simulink model "SF034A_AssiPahFwl"  (R2013b)
settings: Solver=FixedStepDiscrete  SolverMode=SingleTasking  StartTime=0.0  StopTime=1  FixedStep=0.002  RelTol=1e-3
values from neighbouring files (symbols this model uses):
  ARCHGLBPRM_2MILLISEC_SEC_F32 = DataDict.Constant    [SF034A_AssiPahFwl_DataDict.m]
  AssiPahFwlDiRcvr = DataDict.Calibration    [SF034A_AssiPahFwl_DataDict.m]
  AssiPahFwlHysCmpLim = DataDict.Calibration    [SF034A_AssiPahFwl_DataDict.m]
  AssiPahFwlRestoreThd = DataDict.Calibration    [SF034A_AssiPahFwl_DataDict.m]
  BasAssiPahFwlOverLimDiagcFailStep = DataDict.Calibration    [SF034A_AssiPahFwl_DataDict.m]
  BasAssiPahFwlOverLimDiagcPassStep = DataDict.Calibration    [SF034A_AssiPahFwl_DataDict.m]
  BASASSIREACHED_CNT_U08 = DataDict.Constant    [SF034A_AssiPahFwl_DataDict.m]
  HiFrqAssiPahFwlOverLimDiagcFailStep = DataDict.Calibration    [SF034A_AssiPahFwl_DataDict.m]
  HiFrqAssiPahFwlOverLimDiagcPassStep = DataDict.Calibration    [SF034A_AssiPahFwl_DataDict.m]
  HIFRQASSIREACHED_CNT_U08 = DataDict.Constant    [SF034A_AssiPahFwl_DataDict.m]
undefined symbols (not defined in the file or in its folder): MfgEnaSt1, NtcNr1, NtcSts1, sigbuilder_block, SigQlfr1
libraries: simulink x23, Fil x8, NxtrLim x5, FixdToFloat x5, BilnrIntrpnMplX x4, FloatToFixd x4, NxtrAbslt x2, LnrIntrpn x1, NxtrSign x1
(part 2 of 3)

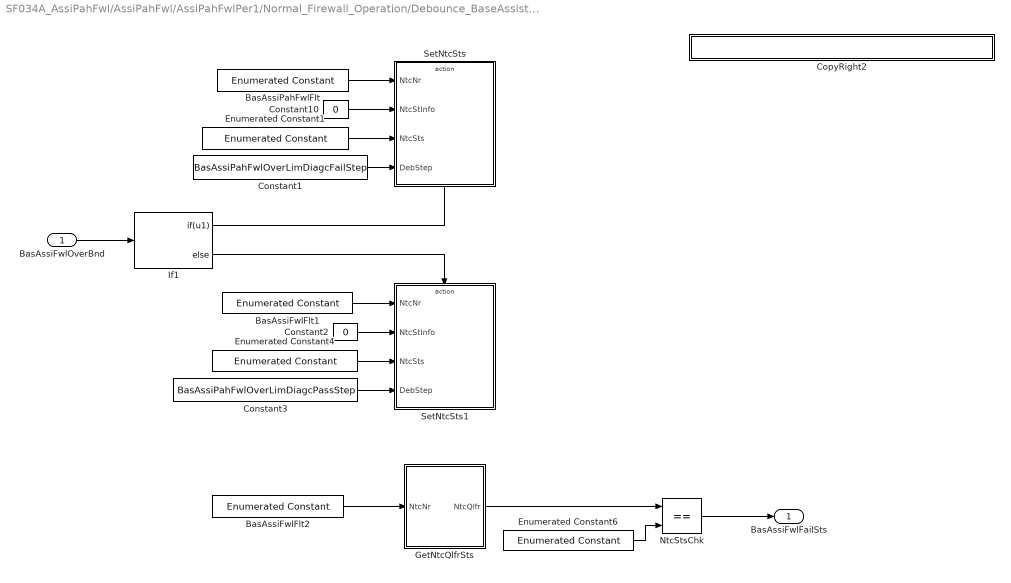
== system SF034A_AssiPahFwl/AssiPahFwl/AssiPahFwlPer1/Normal_Firewall_Operation/Debounce_BaseAssist_Overboundary ==
  BasAssiFwlOverBnd : Inport
  BasAssiFwlFlt1 : simulink/Sources/Enumerated Constant  RequirementInfo={} %GIDa_2f1a8232_f62b_44d9_9001_15c30141b4fe  OutDataTypeStr=Enum: NtcNr1  Value=NtcNr1.NTCNR_0X0D3  SampleTime=inf
  BasAssiFwlFlt2 : simulink/Sources/Enumerated Constant  RequirementInfo={} %GIDa_a465f244_f927_4bf7_a173_7ecad0b77852  OutDataTypeStr=Enum: NtcNr1  Value=NtcNr1.NTCNR_0X0D3  SampleTime=inf
  BasAssiPahFwlFlt : simulink/Sources/Enumerated Constant  RequirementInfo={} %GIDa_799d57aa_42cf_4c29_8873_5e7f7c5dd1ab  OutDataTypeStr=Enum: NtcNr1  Value=NtcNr1.NTCNR_0X0D3  SampleTime=inf
  Constant1 : Constant  Value=BasAssiPahFwlOverLimDiagcFailStep  OutDataTypeStr=uint16
  Constant10 : Constant  Value=0
  Constant2 : Constant  Value=0
  Constant3 : Constant  Value=BasAssiPahFwlOverLimDiagcPassStep  OutDataTypeStr=uint16
  CopyRight2 : Subsystem  Description=|  mask(Copyright Information){none=on}
      | Copyright info block.                                               
      |                                                                     
      | Place copyright information at the top of every subsystem in design.
      mask prompts: none "No parameters"
      mask help: Place copyright information at the top of every subsystem in design.
      mask Display:
      | NxtrConf = 'Nexteer Confidential';
      | 
      | sys = bdroot; %handle for the current model ("system")
      | first = get_param(sys,'Created');
      | first = first(end-3:end);  %year is last four digits
      | 
      | last = get_param(sys,'LastModifiedDate');
      | if isempty(last)
      |     last = datestr(now,'yyyy');
      | else
      |     last = last(end-3:end);
      | end
      | 
      | if strcmp(first,last)
      |     fprintf('%s -- Copyright %s Nexteer',NxtrConf,first)
      | else
      |     fprintf('%s -- %s%s- %s Nexteer',NxtrConf,char(169),first,last)
      | end
  Enumerated Constant1 : simulink/Sources/Enumerated Constant  OutDataTypeStr=Enum: NtcSts1  Value=NtcSts1.NTCSTS_PREFAILD  SampleTime=inf
  Enumerated Constant4 : simulink/Sources/Enumerated Constant  OutDataTypeStr=Enum: NtcSts1  Value=NtcSts1.NTCSTS_PREPASSD  SampleTime=inf
  Enumerated Constant6 : simulink/Sources/Enumerated Constant  RequirementInfo={} %GIDa_ef2938ec_76c4_4b05_b3ba_cb549f411415  OutDataTypeStr=Enum: SigQlfr1  Value=SigQlfr1.SIGQLFR_FAILD  SampleTime=inf
  GetNtcQlfrSts : Subsystem  RequirementInfo={} %GIDa_54fc8d4e_0fa0_427e_9c5d_5132333ac04c  TreatAsAtomicUnit=on  mask(GetNTC){}
      mask help: GetNTC library block
      settings: RTWSystemCode=Inline
  If1 : If  IfExpression=u1
  NtcStsChk : RelationalOperator  RequirementInfo={} %GIDa_8638d8d3_f7fc_4b39_a42c_d5b1eb7d8326  Operator===  OutDataTypeStr=boolean
  SetNtcSts : Subsystem  mask(SetNTC){}
      mask help: SetNTC library block
  SetNtcSts1 : Subsystem  mask(SetNTC){}
      mask help: SetNTC library block
  BasAssiFwlFailSts : Outport
  wires:
  BasAssiFwlOverBnd/1 -> If1/1
  If1/1 -> SetNtcSts/Action
  If1/2 -> SetNtcSts1/Action
  Enumerated Constant1/1 -> SetNtcSts/3(NtcSts)
  Constant1/1 -> SetNtcSts/4(DebStep)
  BasAssiPahFwlFlt/1 -> SetNtcSts/1(NtcNr)
  Constant10/1 -> SetNtcSts/2(NtcStInfo)
  Constant2/1 -> SetNtcSts1/2(NtcStInfo)
  BasAssiFwlFlt1/1 -> SetNtcSts1/1(NtcNr)
  Enumerated Constant4/1 -> SetNtcSts1/3(NtcSts)
  Constant3/1 -> SetNtcSts1/4(DebStep)
  BasAssiFwlFlt2/1 -> GetNtcQlfrSts/1(NtcNr)
  Enumerated Constant6/1 -> NtcStsChk/2
  NtcStsChk/1 -> BasAssiFwlFailSts/1
  GetNtcQlfrSts/1(NtcQlfr) -> NtcStsChk/1

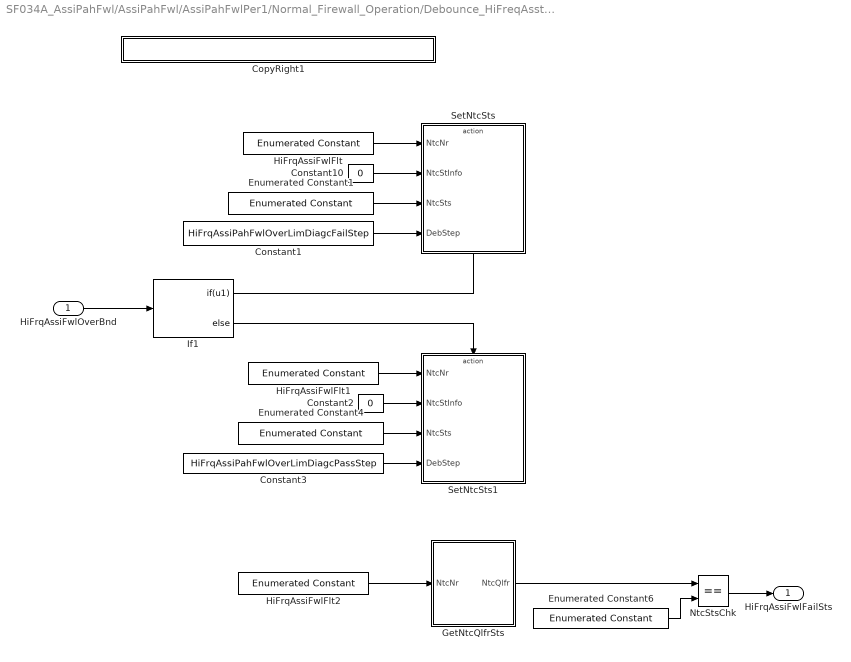
== system SF034A_AssiPahFwl/AssiPahFwl/AssiPahFwlPer1/Normal_Firewall_Operation/Debounce_HiFreqAsst_Overboundary ==
  HiFrqAssiFwlOverBnd : Inport
  Constant1 : Constant  Value=HiFrqAssiPahFwlOverLimDiagcFailStep  OutDataTypeStr=uint16
  Constant10 : Constant  Value=0
  Constant2 : Constant  Value=0
  Constant3 : Constant  Value=HiFrqAssiPahFwlOverLimDiagcPassStep  OutDataTypeStr=uint16
  CopyRight1 : Subsystem  Description=|  mask(Copyright Information){none=on}
      | Copyright info block.                                               
      |                                                                     
      | Place copyright information at the top of every subsystem in design.
      mask prompts: none "No parameters"
      mask help: Place copyright information at the top of every subsystem in design.
      mask Display:
      | NxtrConf = 'Nexteer Confidential';
      | 
      | sys = bdroot; %handle for the current model ("system")
      | first = get_param(sys,'Created');
      | first = first(end-3:end);  %year is last four digits
      | 
      | last = get_param(sys,'LastModifiedDate');
      | if isempty(last)
      |     last = datestr(now,'yyyy');
      | else
      |     last = last(end-3:end);
      | end
      | 
      | if strcmp(first,last)
      |     fprintf('%s -- Copyright %s Nexteer',NxtrConf,first)
      | else
      |     fprintf('%s -- %s%s- %s Nexteer',NxtrConf,char(169),first,last)
      | end
  Enumerated Constant1 : simulink/Sources/Enumerated Constant  OutDataTypeStr=Enum: NtcSts1  Value=NtcSts1.NTCSTS_PREFAILD  SampleTime=inf
  Enumerated Constant4 : simulink/Sources/Enumerated Constant  OutDataTypeStr=Enum: NtcSts1  Value=NtcSts1.NTCSTS_PREPASSD  SampleTime=inf
  Enumerated Constant6 : simulink/Sources/Enumerated Constant  RequirementInfo={} %GIDa_3600cdba_8f0f_4554_a585_bae998e94276  OutDataTypeStr=Enum: SigQlfr1  Value=SigQlfr1.SIGQLFR_FAILD  SampleTime=inf
  GetNtcQlfrSts : Subsystem  RequirementInfo={} %GIDa_f8f859fc_21f7_4c7c_a00d_ec7bd1565e07  TreatAsAtomicUnit=on  mask(GetNTC){}
      mask help: GetNTC library block
      settings: RTWSystemCode=Inline
  HiFrqAssiFwlFlt : simulink/Sources/Enumerated Constant  RequirementInfo={} %GIDa_f02955ec_0115_4e96_8b02_d18904c9c2a9  OutDataTypeStr=Enum: NtcNr1  Value=NtcNr1.NTCNR_0X0D2  SampleTime=inf
  HiFrqAssiFwlFlt1 : simulink/Sources/Enumerated Constant  RequirementInfo={} %GIDa_3a677825_88ef_4104_ad2f_9fc809db66e2  OutDataTypeStr=Enum: NtcNr1  Value=NtcNr1.NTCNR_0X0D2  SampleTime=inf
  HiFrqAssiFwlFlt2 : simulink/Sources/Enumerated Constant  RequirementInfo={} %GIDa_609abb72_ea01_480c_9a92_243e933c8fd0  OutDataTypeStr=Enum: NtcNr1  Value=NtcNr1.NTCNR_0X0D2  SampleTime=inf
  If1 : If  IfExpression=u1
  NtcStsChk : RelationalOperator  RequirementInfo={} %GIDa_02e17ef1_e659_44dd_88b6_676dbdc2e901  Operator===  OutDataTypeStr=boolean
  SetNtcSts : Subsystem  mask(SetNTC){}
      mask help: SetNTC library block
  SetNtcSts1 : Subsystem  mask(SetNTC){}
      mask help: SetNTC library block
  HiFrqAssiFwlFailSts : Outport
  wires:
  HiFrqAssiFwlOverBnd/1 -> If1/1
  If1/1 -> SetNtcSts/Action
  If1/2 -> SetNtcSts1/Action
  Enumerated Constant1/1 -> SetNtcSts/3(NtcSts)
  Constant1/1 -> SetNtcSts/4(DebStep)
  HiFrqAssiFwlFlt/1 -> SetNtcSts/1(NtcNr)
  Constant10/1 -> SetNtcSts/2(NtcStInfo)
  Constant2/1 -> SetNtcSts1/2(NtcStInfo)
  HiFrqAssiFwlFlt1/1 -> SetNtcSts1/1(NtcNr)
  Enumerated Constant4/1 -> SetNtcSts1/3(NtcSts)
  Constant3/1 -> SetNtcSts1/4(DebStep)
  HiFrqAssiFwlFlt2/1 -> GetNtcQlfrSts/1(NtcNr)
  Enumerated Constant6/1 -> NtcStsChk/2
  NtcStsChk/1 -> HiFrqAssiFwlFailSts/1
  GetNtcQlfrSts/1(NtcQlfr) -> NtcStsChk/1

== system SF034A_AssiPahFwl/AssiPahFwl/AssiPahFwlPer1/Normal_Firewall_Operation/Default_AssistDefeat_Firewall ==
  DftAssi : Inport
  Action Port : ActionPort  ActionType=then
  Constant1 : Constant  Value=true  OutDataTypeStr=boolean
      settings: AttributesFormatString=%<OutDataTypeStr>
  Constant3 : Constant  Value=0  OutDataTypeStr=single
      settings: AttributesFormatString=%<OutDataTypeStr>
  CopyRight2 : Subsystem  Description=|  mask(Copyright Information){none=on}
      | Copyright info block.                                               
      |                                                                     
      | Place copyright information at the top of every subsystem in design.
      mask prompts: none "No parameters"
      mask help: Place copyright information at the top of every subsystem in design.
      mask Display:
      | NxtrConf = 'Nexteer Confidential';
      | 
      | sys = bdroot; %handle for the current model ("system")
      | first = get_param(sys,'Created');
      | first = first(end-3:end);  %year is last four digits
      | 
      | last = get_param(sys,'LastModifiedDate');
      | if isempty(last)
      |     last = datestr(now,'yyyy');
      | else
      |     last = last(end-3:end);
      | end
      | 
      | if strcmp(first,last)
      |     fprintf('%s -- Copyright %s Nexteer',NxtrConf,first)
      | else
      |     fprintf('%s -- %s%s- %s Nexteer',NxtrConf,char(169),first,last)
      | end
  CombdAssiDft : Outport
  AssiFwlActvRawDft : Outport  Port=2
  AssiReducedPrfmncDft : Outport  Port=3
  wires:
  DftAssi/1 -> CombdAssiDft/1
  Constant3/1 -> AssiFwlActvRawDft/1
  Constant1/1 -> AssiReducedPrfmncDft/1

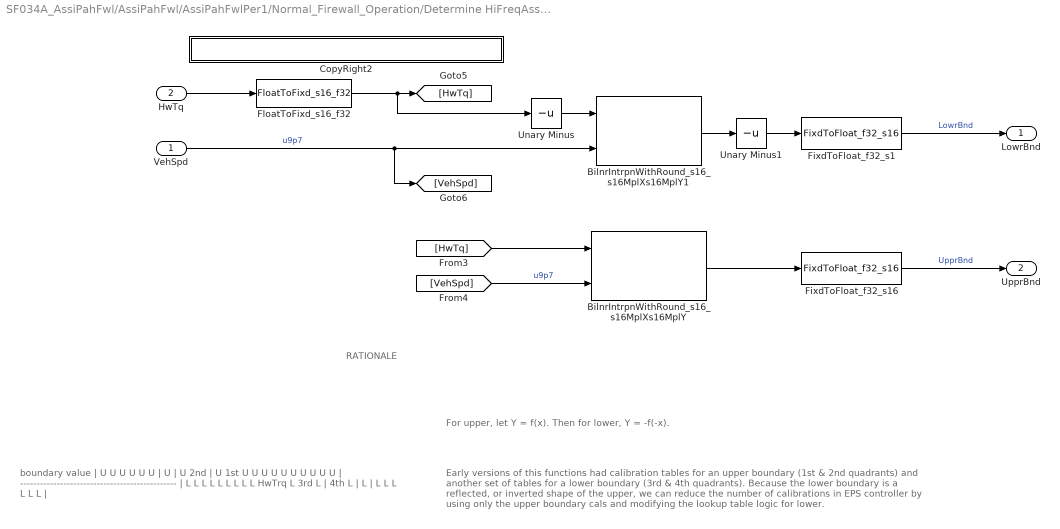
== system SF034A_AssiPahFwl/AssiPahFwl/AssiPahFwlPer1/Normal_Firewall_Operation/Determine HiFreqAsst Boundaries ==
  note: boundary value
      |                    |       U U U U U U
      |                    |     U
      |                    |   U
      |       2nd          | U       1st
      |                    U
      |  U U U U U U U U U |
      | -----------------------------------------------
      |                    | L L L L L L L L L    HwTrq
      |                    L
      |       3rd        L |         4th
      |                L   |
      |              L     |
      |  L L L L L L       |
  note: RATIONALE
  note: Early versions of this functions had calibration tables for an upper boundary (1st & 2nd quadrants)
      | and another set of tables for a lower boundary (3rd & 4th quadrants).  Because the lower boundary
      | is a reflected, or inverted shape of the upper, we can reduce the number of calibrations in EPS
      | controller by using only the upper boundary cals and modifying the lookup table logic for lower.
  note: For upper, let Y = f(x). Then for lower, Y = -f(-x).
  VehSpd : Inport
  HwTq : Inport  Port=2
  BilnrIntrpnWithRound_s16_s16MplXs16MplY : BilnrIntrpnMplX/BilnrIntrpnWithRound_s16_s16MplXs16MplY  MplXTbl=AssiPahFwlUpprLimX  MplYTbl=AssiPahFwlHiFrqUpprLimY  BilnrSelnTbl=AssiPahFwlVehSpd
      settings: AttributesFormatString=Bilnr ( s16MplX , s16MplY )
  BilnrIntrpnWithRound_s16_s16MplXs16MplY1 : BilnrIntrpnMplX/BilnrIntrpnWithRound_s16_s16MplXs16MplY  MplXTbl=AssiPahFwlUpprLimX  MplYTbl=AssiPahFwlHiFrqUpprLimY  BilnrSelnTbl=AssiPahFwlVehSpd
      settings: AttributesFormatString=Bilnr ( s16MplX , s16MplY )
  CopyRight2 : Subsystem  Description=|  mask(Copyright Information){none=on}
      | Copyright info block.                                               
      |                                                                     
      | Place copyright information at the top of every subsystem in design.
      mask prompts: none "No parameters"
      mask help: Place copyright information at the top of every subsystem in design.
      mask Display:
      | NxtrConf = 'Nexteer Confidential';
      | 
      | sys = bdroot; %handle for the current model ("system")
      | first = get_param(sys,'Created');
      | first = first(end-3:end);  %year is last four digits
      | 
      | last = get_param(sys,'LastModifiedDate');
      | if isempty(last)
      |     last = datestr(now,'yyyy');
      | else
      |     last = last(end-3:end);
      | end
      | 
      | if strcmp(first,last)
      |     fprintf('%s -- Copyright %s Nexteer',NxtrConf,first)
      | else
      |     fprintf('%s -- %s%s- %s Nexteer',NxtrConf,char(169),first,last)
      | end
  FixdToFloat_f32_s1 : FixdToFloat/FixdToFloat_f32_s16  Param1=11
  FixdToFloat_f32_s16 : FixdToFloat/FixdToFloat_f32_s16  Param1=11
  FloatToFixd_s16_f32 : FloatToFixd/FloatToFixd_s16_f32  Param1=11
  Unary Minus : UnaryMinus
  Unary Minus1 : UnaryMinus
  LowrBnd : Outport
  UpprBnd : Outport  Port=2
  wires:
  BilnrIntrpnWithRound_s16_s16MplXs16MplY/1 -> FixdToFloat_f32_s16/1
  BilnrIntrpnWithRound_s16_s16MplXs16MplY1/1 -> Unary Minus1/1
  HwTq/1 -> FloatToFixd_s16_f32/1
  FloatToFixd_s16_f32/1 -> Unary Minus/1, [HwTq]
  Unary Minus1/1 -> FixdToFloat_f32_s1/1
  FixdToFloat_f32_s16/1 -> UpprBnd/1  "UpprBnd"
  FixdToFloat_f32_s1/1 -> LowrBnd/1  "LowrBnd"
  [HwTq] -> BilnrIntrpnWithRound_s16_s16MplXs16MplY/1
  [VehSpd] -> BilnrIntrpnWithRound_s16_s16MplXs16MplY/2  "u9p7"
  Unary Minus/1 -> BilnrIntrpnWithRound_s16_s16MplXs16MplY1/1
  VehSpd/1 -> [VehSpd], BilnrIntrpnWithRound_s16_s16MplXs16MplY1/2  "u9p7"

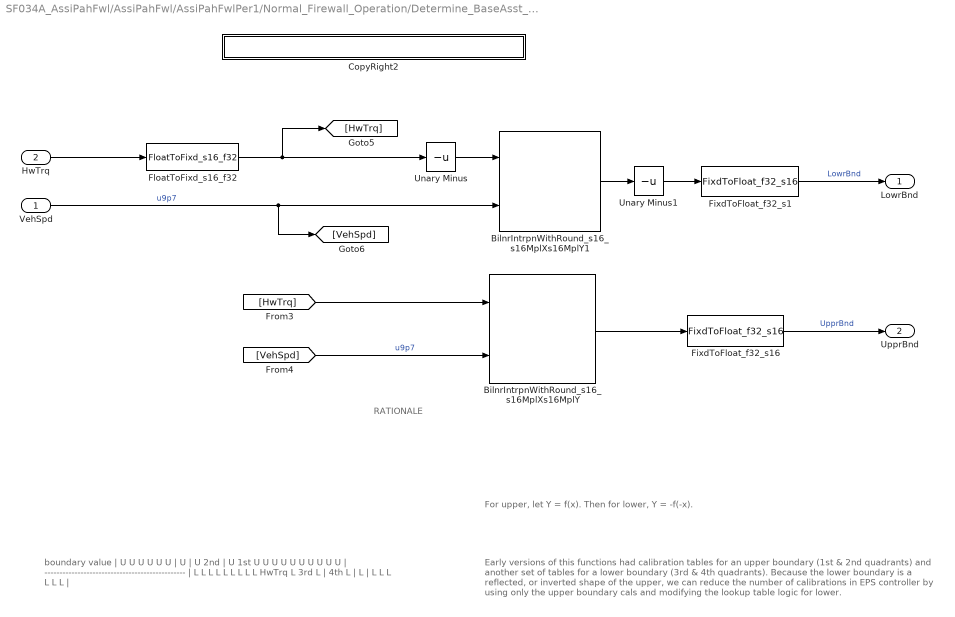
== system SF034A_AssiPahFwl/AssiPahFwl/AssiPahFwlPer1/Normal_Firewall_Operation/Determine_BaseAsst_Boundaries ==
  note: boundary value
      |                    |       U U U U U U
      |                    |     U
      |                    |   U
      |       2nd          | U       1st
      |                    U
      |  U U U U U U U U U |
      | -----------------------------------------------
      |                    | L L L L L L L L L    HwTrq
      |                    L
      |       3rd        L |         4th
      |                L   |
      |              L     |
      |  L L L L L L       |
  note: RATIONALE
  note: Early versions of this functions had calibration tables for an upper boundary (1st & 2nd quadrants)
      | and another set of tables for a lower boundary (3rd & 4th quadrants).  Because the lower boundary
      | is a reflected, or inverted shape of the upper, we can reduce the number of calibrations in EPS
      | controller by using only the upper boundary cals and modifying the lookup table logic for lower.
  note: For upper, let Y = f(x). Then for lower, Y = -f(-x).
  VehSpd : Inport
  HwTrq : Inport  Port=2
  BilnrIntrpnWithRound_s16_s16MplXs16MplY : BilnrIntrpnMplX/BilnrIntrpnWithRound_s16_s16MplXs16MplY  MplXTbl=AssiPahFwlUpprLimX  MplYTbl=AssiPahFwlUpprLimY  BilnrSelnTbl=AssiPahFwlVehSpd
      settings: AttributesFormatString=Bilnr ( s16MplX , s16MplY )
  BilnrIntrpnWithRound_s16_s16MplXs16MplY1 : BilnrIntrpnMplX/BilnrIntrpnWithRound_s16_s16MplXs16MplY  MplXTbl=AssiPahFwlUpprLimX  MplYTbl=AssiPahFwlUpprLimY  BilnrSelnTbl=AssiPahFwlVehSpd
      settings: AttributesFormatString=Bilnr ( s16MplX , s16MplY )
  CopyRight2 : Subsystem  Description=|  mask(Copyright Information){none=on}
      | Copyright info block.                                               
      |                                                                     
      | Place copyright information at the top of every subsystem in design.
      mask prompts: none "No parameters"
      mask help: Place copyright information at the top of every subsystem in design.
      mask Display:
      | NxtrConf = 'Nexteer Confidential';
      | 
      | sys = bdroot; %handle for the current model ("system")
      | first = get_param(sys,'Created');
      | first = first(end-3:end);  %year is last four digits
      | 
      | last = get_param(sys,'LastModifiedDate');
      | if isempty(last)
      |     last = datestr(now,'yyyy');
      | else
      |     last = last(end-3:end);
      | end
      | 
      | if strcmp(first,last)
      |     fprintf('%s -- Copyright %s Nexteer',NxtrConf,first)
      | else
      |     fprintf('%s -- %s%s- %s Nexteer',NxtrConf,char(169),first,last)
      | end
  FixdToFloat_f32_s1 : FixdToFloat/FixdToFloat_f32_s16  Param1=11
  FixdToFloat_f32_s16 : FixdToFloat/FixdToFloat_f32_s16  Param1=11
  FloatToFixd_s16_f32 : FloatToFixd/FloatToFixd_s16_f32  Param1=11
  Unary Minus : UnaryMinus
  Unary Minus1 : UnaryMinus
  LowrBnd : Outport
  UpprBnd : Outport  Port=2
  wires:
  FixdToFloat_f32_s16/1 -> UpprBnd/1  "UpprBnd"
  HwTrq/1 -> FloatToFixd_s16_f32/1
  VehSpd/1 -> BilnrIntrpnWithRound_s16_s16MplXs16MplY1/2, [VehSpd]  "u9p7"
  FloatToFixd_s16_f32/1 -> Unary Minus/1, [HwTrq]
  Unary Minus/1 -> BilnrIntrpnWithRound_s16_s16MplXs16MplY1/1
  Unary Minus1/1 -> FixdToFloat_f32_s1/1
  BilnrIntrpnWithRound_s16_s16MplXs16MplY/1 -> FixdToFloat_f32_s16/1
  FixdToFloat_f32_s1/1 -> LowrBnd/1  "LowrBnd"
  BilnrIntrpnWithRound_s16_s16MplXs16MplY1/1 -> Unary Minus1/1
  [HwTrq] -> BilnrIntrpnWithRound_s16_s16MplXs16MplY/1
  [VehSpd] -> BilnrIntrpnWithRound_s16_s16MplXs16MplY/2  "u9p7"

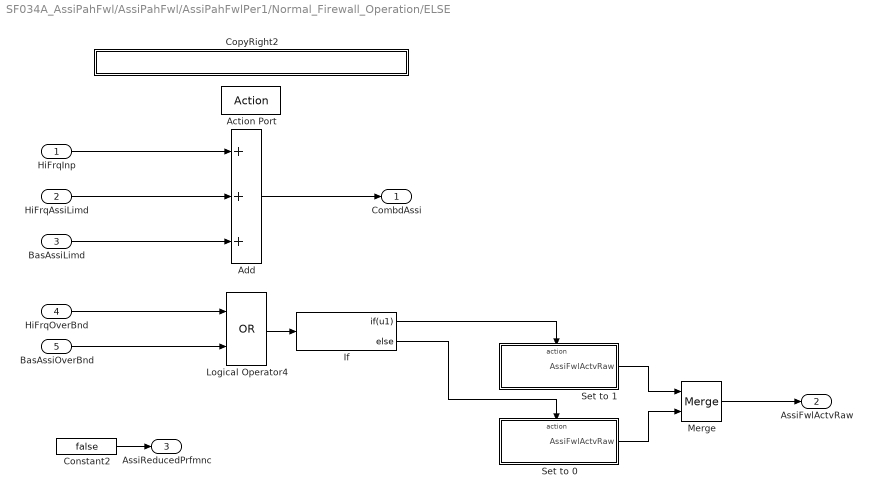
== system SF034A_AssiPahFwl/AssiPahFwl/AssiPahFwlPer1/Normal_Firewall_Operation/ELSE ==
  HiFrqInp : Inport
  HiFrqAssiLimd : Inport  Port=2
  BasAssiLimd : Inport  Port=3
  HiFrqOverBnd : Inport  Port=4
  BasAssiOverBnd : Inport  Port=5
  Action Port : ActionPort  ActionType=else
  Add : Sum  Inputs=+++
  Constant2 : Constant  Value=false  OutDataTypeStr=boolean
      settings: AttributesFormatString=%<OutDataTypeStr>
  CopyRight2 : Subsystem  Description=|  mask(Copyright Information){none=on}
      | Copyright info block.                                               
      |                                                                     
      | Place copyright information at the top of every subsystem in design.
      mask prompts: none "No parameters"
      mask help: Place copyright information at the top of every subsystem in design.
      mask Display:
      | NxtrConf = 'Nexteer Confidential';
      | 
      | sys = bdroot; %handle for the current model ("system")
      | first = get_param(sys,'Created');
      | first = first(end-3:end);  %year is last four digits
      | 
      | last = get_param(sys,'LastModifiedDate');
      | if isempty(last)
      |     last = datestr(now,'yyyy');
      | else
      |     last = last(end-3:end);
      | end
      | 
      | if strcmp(first,last)
      |     fprintf('%s -- Copyright %s Nexteer',NxtrConf,first)
      | else
      |     fprintf('%s -- %s%s- %s Nexteer',NxtrConf,char(169),first,last)
      | end
  If : If  IfExpression=u1
  Logical Operator4 : Logic  Operator=OR  AllPortsSameDT=off  OutDataTypeStr=boolean
  Merge : Merge
  Set to 0 : Subsystem  TreatAsAtomicUnit=on
  Set to 1 : Subsystem  TreatAsAtomicUnit=on
  CombdAssi : Outport
  AssiFwlActvRaw : Outport  Port=2
  AssiReducedPrfmnc : Outport  Port=3
  wires:
  HiFrqInp/1 -> Add/1
  Add/1 -> CombdAssi/1
  HiFrqAssiLimd/1 -> Add/2
  BasAssiLimd/1 -> Add/3
  HiFrqOverBnd/1 -> Logical Operator4/1
  BasAssiOverBnd/1 -> Logical Operator4/2
  Logical Operator4/1 -> If/1
  Constant2/1 -> AssiReducedPrfmnc/1
  If/1 -> Set to 1/Action
  If/2 -> Set to 0/Action
  Set to 1/1(AssiFwlActvRaw) -> Merge/1
  Set to 0/1(AssiFwlActvRaw) -> Merge/2
  Merge/1 -> AssiFwlActvRaw/1

== system SF034A_AssiPahFwl/AssiPahFwl/AssiPahFwlPer1/Normal_Firewall_Operation/Low Pass Filter Boundaries ==
  LowrBnd : Inport
  UpprBnd : Inport  Port=2
  CopyRight2 : Subsystem  Description=|  mask(Copyright Information){none=on}
      | Copyright info block.                                               
      |                                                                     
      | Place copyright information at the top of every subsystem in design.
      mask prompts: none "No parameters"
      mask help: Place copyright information at the top of every subsystem in design.
      mask Display:
      | NxtrConf = 'Nexteer Confidential';
      | 
      | sys = bdroot; %handle for the current model ("system")
      | first = get_param(sys,'Created');
      | first = first(end-3:end);  %year is last four digits
      | 
      | last = get_param(sys,'LastModifiedDate');
      | if isempty(last)
      |     last = datestr(now,'yyyy');
      | else
      |     last = last(end-3:end);
      | end
      | 
      | if strcmp(first,last)
      |     fprintf('%s -- Copyright %s Nexteer',NxtrConf,first)
      | else
      |     fprintf('%s -- %s%s- %s Nexteer',NxtrConf,char(169),first,last)
      | end
  FilLpUpdOutp2 : Fil/FilLpUpdOutp  StVar=LowrLimLpFilStVari
      settings: AttributesFormatString=StVar: %<StVar>
  FilLpUpdOutp3 : Fil/FilLpUpdOutp  StVar=UpprLimLpFilStVari
      settings: AttributesFormatString=StVar: %<StVar>
  LowrBndLpFil : Outport
  UpprBndLpFil : Outport  Port=2
  wires:
  FilLpUpdOutp2/1 -> LowrBndLpFil/1
  FilLpUpdOutp3/1 -> UpprBndLpFil/1
  LowrBnd/1 -> FilLpUpdOutp2/1
  UpprBnd/1 -> FilLpUpdOutp3/1

== system SF034A_AssiPahFwl/AssiPahFwl/AssiPahFwlPer1/Normal_Firewall_Operation/Set_Faults ==
  note: NEXTEER TROUBLE CODE
      | Number  TYPE   Name
      |  0x0C9      F3      NTCNumber.NTC_Num_AssistFWFltMode
  HiFrqAssiFwlReached : Inport  RequirementInfo={} %GIDa_71c3a09e_47b5_4b15_8937_97013ecf90df
  BasAssiFwlReached : Inport  RequirementInfo={} %GIDa_3c1d538b_91e9_4f6c_87ea_f18ffd74aa70  Port=2
  CopyRight2 : Subsystem  Description=|  mask(Copyright Information){none=on}
      | Copyright info block.                                               
      |                                                                     
      | Place copyright information at the top of every subsystem in design.
      mask prompts: none "No parameters"
      mask help: Place copyright information at the top of every subsystem in design.
      mask Display:
      | NxtrConf = 'Nexteer Confidential';
      | 
      | sys = bdroot; %handle for the current model ("system")
      | first = get_param(sys,'Created');
      | first = first(end-3:end);  %year is last four digits
      | 
      | last = get_param(sys,'LastModifiedDate');
      | if isempty(last)
      |     last = datestr(now,'yyyy');
      | else
      |     last = last(end-3:end);
      | end
      | 
      | if strcmp(first,last)
      |     fprintf('%s -- Copyright %s Nexteer',NxtrConf,first)
      | else
      |     fprintf('%s -- %s%s- %s Nexteer',NxtrConf,char(169),first,last)
      | end
  If : If  IfExpression=u1  ShowElse=off
  Logical Operator : Logic  Operator=OR  AllPortsSameDT=off  OutDataTypeStr=boolean
  Set AssiFwlFlt : Subsystem  TreatAsAtomicUnit=on
  wires:
  Logical Operator/1 -> If/1
  HiFrqAssiFwlReached/1 -> Set AssiFwlFlt/1(HiFrqAssiFwlReached), Logical Operator/1
  BasAssiFwlReached/1 -> Set AssiFwlFlt/2(BasAssiFwlReached), Logical Operator/2
  If/1 -> Set AssiFwlFlt/Action

== system SF034A_AssiPahFwl/AssiPahFwl/AssiPahFwlInit1/AssiFwlFltMode/SetNtcSts/CopyRight2 ==

== system SF034A_AssiPahFwl/AssiPahFwl/AssiPahFwlInit1/BaseAssistFwlReached/SetNtcSts/CopyRight2 ==

== system SF034A_AssiPahFwl/AssiPahFwl/AssiPahFwlInit1/HiFrqAssiFwlReached/SetNtcSts/CopyRight2 ==

== system SF034A_AssiPahFwl/AssiPahFwl/AssiPahFwlPer1/Normal_Firewall_Operation/Debounce_BaseAssist_Overboundary/CopyRight2 ==

== system SF034A_AssiPahFwl/AssiPahFwl/AssiPahFwlPer1/Normal_Firewall_Operation/Debounce_BaseAssist_Overboundary/GetNtcQlfrSts ==
  NtcNr : Inport
  CopyRight2 : Subsystem  Description=|  mask(Copyright Information){none=on}
      | Copyright info block.                                               
      |                                                                     
      | Place copyright information at the top of every subsystem in design.
      mask prompts: none "No parameters"
      mask help: Place copyright information at the top of every subsystem in design.
      mask Display:
      | NxtrConf = 'Nexteer Confidential';
      | 
      | sys = bdroot; %handle for the current model ("system")
      | first = get_param(sys,'Created');
      | first = first(end-3:end);  %year is last four digits
      | 
      | last = get_param(sys,'LastModifiedDate');
      | if isempty(last)
      |     last = datestr(now,'yyyy');
      | else
      |     last = last(end-3:end);
      | end
      | 
      | if strcmp(first,last)
      |     fprintf('%s -- Copyright %s Nexteer',NxtrConf,first)
      | else
      |     fprintf('%s -- %s%s- %s Nexteer',NxtrConf,char(169),first,last)
      | end
  Data Store Read : DataStoreRead  DataStoreName=Ntc0x0D3Qlfr
  Terminator : Terminator
  NtcQlfr : Outport
  wires:
  Data Store Read/1 -> NtcQlfr/1
  NtcNr/1 -> Terminator/1

== system SF034A_AssiPahFwl/AssiPahFwl/AssiPahFwlPer1/Normal_Firewall_Operation/Debounce_BaseAssist_Overboundary/SetNtcSts ==
  NtcNr : Inport
  NtcStInfo : Inport  Port=2
  NtcSts : Inport  Port=3
  DebStep : Inport  Port=4
  CallDiagMgr : ActionPort  ActionType=then
  SetNtcSts : Subsystem  RequirementInfo={} %GIDa_7903117e_c9ff_4bda_a70f_dd3a2a192cde  TreatAsAtomicUnit=on
      settings: RTWSystemCode=Inline
  wires:
  NtcStInfo/1 -> SetNtcSts/2(NtcStInfo)
  DebStep/1 -> SetNtcSts/4(DebStep)
  NtcSts/1 -> SetNtcSts/3(NtcSts)
  NtcNr/1 -> SetNtcSts/1(NtcNr)  "NtcNr"

== system SF034A_AssiPahFwl/AssiPahFwl/AssiPahFwlPer1/Normal_Firewall_Operation/Debounce_BaseAssist_Overboundary/SetNtcSts1 ==
  NtcNr : Inport
  NtcStInfo : Inport  Port=2
  NtcSts : Inport  Port=3
  DebStep : Inport  Port=4
  CallDiagMgr : ActionPort  ActionType=else
  SetNtcSts : Subsystem  RequirementInfo={} %GIDa_56e3945b_2fe9_4d42_adb2_3064db088301  TreatAsAtomicUnit=on
      settings: RTWSystemCode=Inline
  wires:
  NtcNr/1 -> SetNtcSts/1(NtcNr)  "NtcNr"
  NtcSts/1 -> SetNtcSts/3(NtcSts)
  DebStep/1 -> SetNtcSts/4(DebStep)
  NtcStInfo/1 -> SetNtcSts/2(NtcStInfo)

== system SF034A_AssiPahFwl/AssiPahFwl/AssiPahFwlPer1/Normal_Firewall_Operation/Debounce_HiFreqAsst_Overboundary/CopyRight1 ==

== system SF034A_AssiPahFwl/AssiPahFwl/AssiPahFwlPer1/Normal_Firewall_Operation/Debounce_HiFreqAsst_Overboundary/GetNtcQlfrSts ==
  NtcNr : Inport
  CopyRight2 : Subsystem  Description=|  mask(Copyright Information){none=on}
      | Copyright info block.                                               
      |                                                                     
      | Place copyright information at the top of every subsystem in design.
      mask prompts: none "No parameters"
      mask help: Place copyright information at the top of every subsystem in design.
      mask Display:
      | NxtrConf = 'Nexteer Confidential';
      | 
      | sys = bdroot; %handle for the current model ("system")
      | first = get_param(sys,'Created');
      | first = first(end-3:end);  %year is last four digits
      | 
      | last = get_param(sys,'LastModifiedDate');
      | if isempty(last)
      |     last = datestr(now,'yyyy');
      | else
      |     last = last(end-3:end);
      | end
      | 
      | if strcmp(first,last)
      |     fprintf('%s -- Copyright %s Nexteer',NxtrConf,first)
      | else
      |     fprintf('%s -- %s%s- %s Nexteer',NxtrConf,char(169),first,last)
      | end
  Data Store Read : DataStoreRead  DataStoreName=Ntc0x0D2Qlfr
  Terminator : Terminator
  NtcQlfr : Outport
  wires:
  Data Store Read/1 -> NtcQlfr/1
  NtcNr/1 -> Terminator/1

== system SF034A_AssiPahFwl/AssiPahFwl/AssiPahFwlPer1/Normal_Firewall_Operation/Debounce_HiFreqAsst_Overboundary/SetNtcSts ==
  NtcNr : Inport
  NtcStInfo : Inport  Port=2
  NtcSts : Inport  Port=3
  DebStep : Inport  Port=4
  CallDiagMgr : ActionPort  ActionType=then
  SetNtcSts : Subsystem  RequirementInfo={} %GIDa_c97743af_c8af_47cc_bfa4_4819e3223fd6  TreatAsAtomicUnit=on
      settings: RTWSystemCode=Inline
  wires:
  NtcStInfo/1 -> SetNtcSts/2(NtcStInfo)
  DebStep/1 -> SetNtcSts/4(DebStep)
  NtcSts/1 -> SetNtcSts/3(NtcSts)
  NtcNr/1 -> SetNtcSts/1(NtcNr)  "NtcNr"

== system SF034A_AssiPahFwl/AssiPahFwl/AssiPahFwlPer1/Normal_Firewall_Operation/Debounce_HiFreqAsst_Overboundary/SetNtcSts1 ==
  NtcNr : Inport
  NtcStInfo : Inport  Port=2
  NtcSts : Inport  Port=3
  DebStep : Inport  Port=4
  CallDiagMgr : ActionPort  ActionType=else
  SetNtcSts : Subsystem  RequirementInfo={} %GIDa_eac91af3_404c_49ff_bb66_429add3c1ebb  TreatAsAtomicUnit=on
      settings: RTWSystemCode=Inline
  wires:
  NtcNr/1 -> SetNtcSts/1(NtcNr)  "NtcNr"
  NtcSts/1 -> SetNtcSts/3(NtcSts)
  DebStep/1 -> SetNtcSts/4(DebStep)
  NtcStInfo/1 -> SetNtcSts/2(NtcStInfo)

== system SF034A_AssiPahFwl/AssiPahFwl/AssiPahFwlPer1/Normal_Firewall_Operation/Default_AssistDefeat_Firewall/CopyRight2 ==

== system SF034A_AssiPahFwl/AssiPahFwl/AssiPahFwlPer1/Normal_Firewall_Operation/Determine HiFreqAsst Boundaries/CopyRight2 ==

== system SF034A_AssiPahFwl/AssiPahFwl/AssiPahFwlPer1/Normal_Firewall_Operation/Determine_BaseAsst_Boundaries/CopyRight2 ==

== system SF034A_AssiPahFwl/AssiPahFwl/AssiPahFwlPer1/Normal_Firewall_Operation/ELSE/CopyRight2 ==

== system SF034A_AssiPahFwl/AssiPahFwl/AssiPahFwlPer1/Normal_Firewall_Operation/ELSE/Set to 0 ==
  Action Port : ActionPort  ActionType=else
  Constant : Constant  Value=0  OutDataTypeStr=single
      settings: AttributesFormatString=%<OutDataTypeStr>
  AssiFwlActvRaw : Outport
  wires:
  Constant/1 -> AssiFwlActvRaw/1

== system SF034A_AssiPahFwl/AssiPahFwl/AssiPahFwlPer1/Normal_Firewall_Operation/ELSE/Set to 1 ==
  Action Port : ActionPort  ActionType=then
  Constant : Constant  OutDataTypeStr=single
      settings: AttributesFormatString=%<OutDataTypeStr>
  AssiFwlActvRaw : Outport
  wires:
  Constant/1 -> AssiFwlActvRaw/1

== system SF034A_AssiPahFwl/AssiPahFwl/AssiPahFwlPer1/Normal_Firewall_Operation/Low Pass Filter Boundaries/CopyRight2 ==

== system SF034A_AssiPahFwl/AssiPahFwl/AssiPahFwlPer1/Normal_Firewall_Operation/Set_Faults/CopyRight2 ==

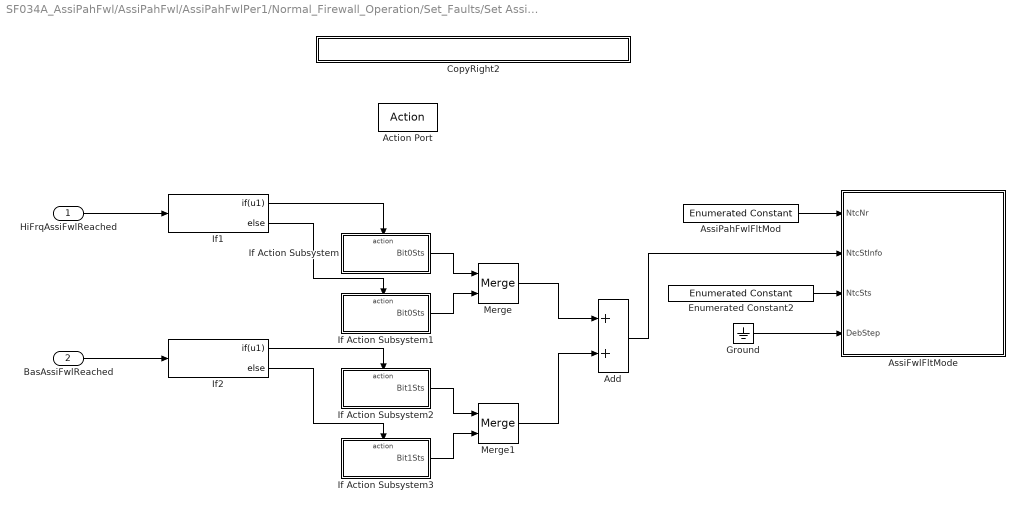
== system SF034A_AssiPahFwl/AssiPahFwl/AssiPahFwlPer1/Normal_Firewall_Operation/Set_Faults/Set AssiFwlFlt ==
  HiFrqAssiFwlReached : Inport
  BasAssiFwlReached : Inport  Port=2
  Action Port : ActionPort  ActionType=then
  Add : Sum
  AssiFwlFltMode : Subsystem  RequirementInfo={} %GIDa_d0a632f1_979d_4e67_880d_9dd9f353dc2a  mask(SetNTC){}
      mask help: SetNTC library block
  AssiPahFwlFltMod : simulink/Sources/Enumerated Constant  RequirementInfo={} %GIDa_ef64cbe5_a81a_4768_aa55_c39d1941ff83  OutDataTypeStr=Enum: NtcNr1  Value=NtcNr1.NTCNR_0X0C9  SampleTime=inf
  CopyRight2 : Subsystem  Description=|  mask(Copyright Information){none=on}
      | Copyright info block.                                               
      |                                                                     
      | Place copyright information at the top of every subsystem in design.
      mask prompts: none "No parameters"
      mask help: Place copyright information at the top of every subsystem in design.
      mask Display:
      | NxtrConf = 'Nexteer Confidential';
      | 
      | sys = bdroot; %handle for the current model ("system")
      | first = get_param(sys,'Created');
      | first = first(end-3:end);  %year is last four digits
      | 
      | last = get_param(sys,'LastModifiedDate');
      | if isempty(last)
      |     last = datestr(now,'yyyy');
      | else
      |     last = last(end-3:end);
      | end
      | 
      | if strcmp(first,last)
      |     fprintf('%s -- Copyright %s Nexteer',NxtrConf,first)
      | else
      |     fprintf('%s -- %s%s- %s Nexteer',NxtrConf,char(169),first,last)
      | end
  Enumerated Constant2 : simulink/Sources/Enumerated Constant  RequirementInfo={} %GIDa_dbcba8aa_b400_445c_8ab9_a0f3a83a58a9  OutDataTypeStr=Enum: NtcSts1  Value=NtcSts1.NTCSTS_FAILD  SampleTime=inf
  Ground : Ground
  If Action Subsystem : Subsystem  TreatAsAtomicUnit=on
  If Action Subsystem1 : Subsystem  TreatAsAtomicUnit=on
  If Action Subsystem2 : Subsystem  TreatAsAtomicUnit=on
  If Action Subsystem3 : Subsystem  TreatAsAtomicUnit=on
  If1 : If  IfExpression=u1
  If2 : If  IfExpression=u1
  Merge : Merge
  Merge1 : Merge
  wires:
  AssiPahFwlFltMod/1 -> AssiFwlFltMode/1(NtcNr)
  Ground/1 -> AssiFwlFltMode/4(DebStep)
  Enumerated Constant2/1 -> AssiFwlFltMode/3(NtcSts)
  HiFrqAssiFwlReached/1 -> If1/1
  BasAssiFwlReached/1 -> If2/1
  If1/1 -> If Action Subsystem/Action
  If1/2 -> If Action Subsystem1/Action
  If2/1 -> If Action Subsystem2/Action
  If2/2 -> If Action Subsystem3/Action
  Add/1 -> AssiFwlFltMode/2(NtcStInfo)
  If Action Subsystem/1(Bit0Sts) -> Merge/1
  If Action Subsystem1/1(Bit0Sts) -> Merge/2
  If Action Subsystem2/1(Bit1Sts) -> Merge1/1
  If Action Subsystem3/1(Bit1Sts) -> Merge1/2
  Merge/1 -> Add/1
  Merge1/1 -> Add/2

== system SF034A_AssiPahFwl/AssiPahFwl/AssiPahFwlPer1/Normal_Firewall_Operation/Debounce_BaseAssist_Overboundary/GetNtcQlfrSts/CopyRight2 ==

== system SF034A_AssiPahFwl/AssiPahFwl/AssiPahFwlPer1/Normal_Firewall_Operation/Debounce_BaseAssist_Overboundary/SetNtcSts/SetNtcSts ==
  note: Note:
      |
      | - "ISO Fault Debounce Design" Simulink block intent to use here for Simulation purpose only. Do not Code this block
  NtcNr : Inport
  NtcStInfo : Inport  Port=2
  NtcSts : Inport  Port=3
  DebStep : Inport  Port=4
  CopyRight2 : Subsystem  Description=|  mask(Copyright Information){none=on}
      | Copyright info block.                                               
      |                                                                     
      | Place copyright information at the top of every subsystem in design.
      mask prompts: none "No parameters"
      mask help: Place copyright information at the top of every subsystem in design.
      mask Display:
      | NxtrConf = 'Nexteer Confidential';
      | 
      | sys = bdroot; %handle for the current model ("system")
      | first = get_param(sys,'Created');
      | first = first(end-3:end);  %year is last four digits
      | 
      | last = get_param(sys,'LastModifiedDate');
      | if isempty(last)
      |     last = datestr(now,'yyyy');
      | else
      |     last = last(end-3:end);
      | end
      | 
      | if strcmp(first,last)
      |     fprintf('%s -- Copyright %s Nexteer',NxtrConf,first)
      | else
      |     fprintf('%s -- %s%s- %s Nexteer',NxtrConf,char(169),first,last)
      | end
  Data Store Write : DataStoreWrite  DataStoreName=Ntc0x0D3Qlfr
  Data Type Conversion : DataTypeConversion  OutDataTypeStr=Enum: SigQlfr1
  Ground : Ground
  ISO Fault Debounce Design : Stateflow chart  TreatAsAtomicUnit=on
      settings: AttributesFormatString=|
      | Simulation Purpose Only.
      | Do Not Code this block
      | Diagnostic Manager Owns this requirement
  Terminator : Terminator
  Terminator1 : Terminator
  wires:
  Ground/1 -> ISO Fault Debounce Design/3(SvcClr)
  ISO Fault Debounce Design/1(Qualifier) -> Data Type Conversion/1
  DebStep/1 -> ISO Fault Debounce Design/2(DebStep)
  NtcSts/1 -> ISO Fault Debounce Design/1(NtcSts)
  NtcNr/1 -> Terminator/1
  NtcStInfo/1 -> Terminator1/1
  Data Type Conversion/1 -> Data Store Write/1

== system SF034A_AssiPahFwl/AssiPahFwl/AssiPahFwlPer1/Normal_Firewall_Operation/Debounce_BaseAssist_Overboundary/SetNtcSts1/SetNtcSts ==
  note: Note:
      |
      | - "ISO Fault Debounce Design" Simulink block intent to use here for Simulation purpose only. Do not Code this block
  NtcNr : Inport
  NtcStInfo : Inport  Port=2
  NtcSts : Inport  Port=3
  DebStep : Inport  Port=4
  CopyRight2 : Subsystem  Description=|  mask(Copyright Information){none=on}
      | Copyright info block.                                               
      |                                                                     
      | Place copyright information at the top of every subsystem in design.
      mask prompts: none "No parameters"
      mask help: Place copyright information at the top of every subsystem in design.
      mask Display:
      | NxtrConf = 'Nexteer Confidential';
      | 
      | sys = bdroot; %handle for the current model ("system")
      | first = get_param(sys,'Created');
      | first = first(end-3:end);  %year is last four digits
      | 
      | last = get_param(sys,'LastModifiedDate');
      | if isempty(last)
      |     last = datestr(now,'yyyy');
      | else
      |     last = last(end-3:end);
      | end
      | 
      | if strcmp(first,last)
      |     fprintf('%s -- Copyright %s Nexteer',NxtrConf,first)
      | else
      |     fprintf('%s -- %s%s- %s Nexteer',NxtrConf,char(169),first,last)
      | end
  Data Store Write : DataStoreWrite  DataStoreName=Ntc0x0D3Qlfr
  Data Type Conversion : DataTypeConversion  OutDataTypeStr=Enum: SigQlfr1
  Ground : Ground
  ISO Fault Debounce Design : Stateflow chart  TreatAsAtomicUnit=on
      settings: AttributesFormatString=|
      | Simulation Purpose Only.
      | Do Not Code this block
      | Diagnostic Manager Owns this requirement
  Terminator : Terminator
  Terminator1 : Terminator
  wires:
  NtcStInfo/1 -> Terminator1/1
  NtcNr/1 -> Terminator/1
  NtcSts/1 -> ISO Fault Debounce Design/1(NtcSts)
  DebStep/1 -> ISO Fault Debounce Design/2(DebStep)
  ISO Fault Debounce Design/1(Qualifier) -> Data Type Conversion/1
  Ground/1 -> ISO Fault Debounce Design/3(SvcClr)
  Data Type Conversion/1 -> Data Store Write/1

== system SF034A_AssiPahFwl/AssiPahFwl/AssiPahFwlPer1/Normal_Firewall_Operation/Debounce_HiFreqAsst_Overboundary/GetNtcQlfrSts/CopyRight2 ==

== system SF034A_AssiPahFwl/AssiPahFwl/AssiPahFwlPer1/Normal_Firewall_Operation/Debounce_HiFreqAsst_Overboundary/SetNtcSts/SetNtcSts ==
  note: Note:
      |
      | - "ISO Fault Debounce Design" Simulink block intent to use here for Simulation purpose only. Do not Code this block
  NtcNr : Inport
  NtcStInfo : Inport  Port=2
  NtcSts : Inport  Port=3
  DebStep : Inport  Port=4
  CopyRight2 : Subsystem  Description=|  mask(Copyright Information){none=on}
      | Copyright info block.                                               
      |                                                                     
      | Place copyright information at the top of every subsystem in design.
      mask prompts: none "No parameters"
      mask help: Place copyright information at the top of every subsystem in design.
      mask Display:
      | NxtrConf = 'Nexteer Confidential';
      | 
      | sys = bdroot; %handle for the current model ("system")
      | first = get_param(sys,'Created');
      | first = first(end-3:end);  %year is last four digits
      | 
      | last = get_param(sys,'LastModifiedDate');
      | if isempty(last)
      |     last = datestr(now,'yyyy');
      | else
      |     last = last(end-3:end);
      | end
      | 
      | if strcmp(first,last)
      |     fprintf('%s -- Copyright %s Nexteer',NxtrConf,first)
      | else
      |     fprintf('%s -- %s%s- %s Nexteer',NxtrConf,char(169),first,last)
      | end
  Data Store Write : DataStoreWrite  DataStoreName=Ntc0x0D2Qlfr
  Data Type Conversion : DataTypeConversion  OutDataTypeStr=Enum: SigQlfr1
  Ground : Ground
  ISO Fault Debounce Design : Stateflow chart  TreatAsAtomicUnit=on
      settings: AttributesFormatString=|
      | Simulation Purpose Only.
      | Do Not Code this block
      | Diagnostic Manager Owns this requirement
  Terminator : Terminator
  Terminator1 : Terminator
  wires:
  Ground/1 -> ISO Fault Debounce Design/3(SvcClr)
  ISO Fault Debounce Design/1(Qualifier) -> Data Type Conversion/1
  DebStep/1 -> ISO Fault Debounce Design/2(DebStep)
  NtcSts/1 -> ISO Fault Debounce Design/1(NtcSts)
  NtcNr/1 -> Terminator/1
  NtcStInfo/1 -> Terminator1/1
  Data Type Conversion/1 -> Data Store Write/1

== system SF034A_AssiPahFwl/AssiPahFwl/AssiPahFwlPer1/Normal_Firewall_Operation/Debounce_HiFreqAsst_Overboundary/SetNtcSts1/SetNtcSts ==
  note: Note:
      |
      | - "ISO Fault Debounce Design" Simulink block intent to use here for Simulation purpose only. Do not Code this block
  NtcNr : Inport
  NtcStInfo : Inport  Port=2
  NtcSts : Inport  Port=3
  DebStep : Inport  Port=4
  CopyRight2 : Subsystem  Description=|  mask(Copyright Information){none=on}
      | Copyright info block.                                               
      |                                                                     
      | Place copyright information at the top of every subsystem in design.
      mask prompts: none "No parameters"
      mask help: Place copyright information at the top of every subsystem in design.
      mask Display:
      | NxtrConf = 'Nexteer Confidential';
      | 
      | sys = bdroot; %handle for the current model ("system")
      | first = get_param(sys,'Created');
      | first = first(end-3:end);  %year is last four digits
      | 
      | last = get_param(sys,'LastModifiedDate');
      | if isempty(last)
      |     last = datestr(now,'yyyy');
      | else
      |     last = last(end-3:end);
      | end
      | 
      | if strcmp(first,last)
      |     fprintf('%s -- Copyright %s Nexteer',NxtrConf,first)
      | else
      |     fprintf('%s -- %s%s- %s Nexteer',NxtrConf,char(169),first,last)
      | end
  Data Store Write : DataStoreWrite  DataStoreName=Ntc0x0D2Qlfr
  Data Type Conversion : DataTypeConversion  OutDataTypeStr=Enum: SigQlfr1
  Ground : Ground
  ISO Fault Debounce Design : Stateflow chart  TreatAsAtomicUnit=on
      settings: AttributesFormatString=|
      | Simulation Purpose Only.
      | Do Not Code this block
      | Diagnostic Manager Owns this requirement
  Terminator : Terminator
  Terminator1 : Terminator
  wires:
  NtcStInfo/1 -> Terminator1/1
  NtcNr/1 -> Terminator/1
  NtcSts/1 -> ISO Fault Debounce Design/1(NtcSts)
  DebStep/1 -> ISO Fault Debounce Design/2(DebStep)
  ISO Fault Debounce Design/1(Qualifier) -> Data Type Conversion/1
  Ground/1 -> ISO Fault Debounce Design/3(SvcClr)
  Data Type Conversion/1 -> Data Store Write/1

== system SF034A_AssiPahFwl/AssiPahFwl/AssiPahFwlPer1/Normal_Firewall_Operation/Set_Faults/Set AssiFwlFlt/AssiFwlFltMode ==
  NtcNr : Inport
  NtcStInfo : Inport  Port=2
  NtcSts : Inport  Port=3
  DebStep : Inport  Port=4
  CopyRight2 : Subsystem  Description=|  mask(Copyright Information){none=on}
      | Copyright info block.                                               
      |                                                                     
      | Place copyright information at the top of every subsystem in design.
      mask prompts: none "No parameters"
      mask help: Place copyright information at the top of every subsystem in design.
      mask Display:
      | NxtrConf = 'Nexteer Confidential';
      | 
      | sys = bdroot; %handle for the current model ("system")
      | first = get_param(sys,'Created');
      | first = first(end-3:end);  %year is last four digits
      | 
      | last = get_param(sys,'LastModifiedDate');
      | if isempty(last)
      |     last = datestr(now,'yyyy');
      | else
      |     last = last(end-3:end);
      | end
      | 
      | if strcmp(first,last)
      |     fprintf('%s -- Copyright %s Nexteer',NxtrConf,first)
      | else
      |     fprintf('%s -- %s%s- %s Nexteer',NxtrConf,char(169),first,last)
      | end
  SetNtcSts : Subsystem  RequirementInfo={} %GIDa_ba0f6a2a_09f3_49ff_aa94_a81bdbdb8fe4  TreatAsAtomicUnit=on
      settings: RTWSystemCode=Inline
  wires:
  NtcStInfo/1 -> SetNtcSts/2(NtcStInfo)
  DebStep/1 -> SetNtcSts/4(DebStep)
  NtcSts/1 -> SetNtcSts/3(NtcSts)
  NtcNr/1 -> SetNtcSts/1(NtcNr)  "NtcNr"

== system SF034A_AssiPahFwl/AssiPahFwl/AssiPahFwlPer1/Normal_Firewall_Operation/Set_Faults/Set AssiFwlFlt/CopyRight2 ==

== system SF034A_AssiPahFwl/AssiPahFwl/AssiPahFwlPer1/Normal_Firewall_Operation/Set_Faults/Set AssiFwlFlt/If Action Subsystem ==
  Action Port : ActionPort  ActionType=then
  Constant : Constant  Value=HIFRQASSIREACHED_CNT_U08
  Constant1 : Constant  OutDataTypeStr=uint8
      settings: AttributesFormatString=%<OutDataTypeStr>
  CopyRight2 : Subsystem  Description=|  mask(Copyright Information){none=on}
      | Copyright info block.                                               
      |                                                                     
      | Place copyright information at the top of every subsystem in design.
      mask prompts: none "No parameters"
      mask help: Place copyright information at the top of every subsystem in design.
      mask Display:
      | NxtrConf = 'Nexteer Confidential';
      | 
      | sys = bdroot; %handle for the current model ("system")
      | first = get_param(sys,'Created');
      | first = first(end-3:end);  %year is last four digits
      | 
      | last = get_param(sys,'LastModifiedDate');
      | if isempty(last)
      |     last = datestr(now,'yyyy');
      | else
      |     last = last(end-3:end);
      | end
      | 
      | if strcmp(first,last)
      |     fprintf('%s -- Copyright %s Nexteer',NxtrConf,first)
      | else
      |     fprintf('%s -- %s%s- %s Nexteer',NxtrConf,char(169),first,last)
      | end
  Product1 : Product
  Bit0Sts : Outport
  wires:
  Constant/1 -> Product1/2
  Constant1/1 -> Product1/1
  Product1/1 -> Bit0Sts/1

== system SF034A_AssiPahFwl/AssiPahFwl/AssiPahFwlPer1/Normal_Firewall_Operation/Set_Faults/Set AssiFwlFlt/If Action Subsystem1 ==
  Action Port : ActionPort  ActionType=else
  Constant : Constant  Value=HIFRQASSIREACHED_CNT_U08
  Constant1 : Constant  Value=0  OutDataTypeStr=uint8
      settings: AttributesFormatString=%<OutDataTypeStr>
  CopyRight2 : Subsystem  Description=|  mask(Copyright Information){none=on}
      | Copyright info block.                                               
      |                                                                     
      | Place copyright information at the top of every subsystem in design.
      mask prompts: none "No parameters"
      mask help: Place copyright information at the top of every subsystem in design.
      mask Display:
      | NxtrConf = 'Nexteer Confidential';
      | 
      | sys = bdroot; %handle for the current model ("system")
      | first = get_param(sys,'Created');
      | first = first(end-3:end);  %year is last four digits
      | 
      | last = get_param(sys,'LastModifiedDate');
      | if isempty(last)
      |     last = datestr(now,'yyyy');
      | else
      |     last = last(end-3:end);
      | end
      | 
      | if strcmp(first,last)
      |     fprintf('%s -- Copyright %s Nexteer',NxtrConf,first)
      | else
      |     fprintf('%s -- %s%s- %s Nexteer',NxtrConf,char(169),first,last)
      | end
  Product1 : Product
  Bit0Sts : Outport
  wires:
  Constant/1 -> Product1/2
  Constant1/1 -> Product1/1
  Product1/1 -> Bit0Sts/1

== system SF034A_AssiPahFwl/AssiPahFwl/AssiPahFwlPer1/Normal_Firewall_Operation/Set_Faults/Set AssiFwlFlt/If Action Subsystem2 ==
  Action Port : ActionPort  ActionType=then
  Constant1 : Constant  OutDataTypeStr=uint8
      settings: AttributesFormatString=%<OutDataTypeStr>
  Constant2 : Constant  Value=BASASSIREACHED_CNT_U08
  CopyRight2 : Subsystem  Description=|  mask(Copyright Information){none=on}
      | Copyright info block.                                               
      |                                                                     
      | Place copyright information at the top of every subsystem in design.
      mask prompts: none "No parameters"
      mask help: Place copyright information at the top of every subsystem in design.
      mask Display:
      | NxtrConf = 'Nexteer Confidential';
      | 
      | sys = bdroot; %handle for the current model ("system")
      | first = get_param(sys,'Created');
      | first = first(end-3:end);  %year is last four digits
      | 
      | last = get_param(sys,'LastModifiedDate');
      | if isempty(last)
      |     last = datestr(now,'yyyy');
      | else
      |     last = last(end-3:end);
      | end
      | 
      | if strcmp(first,last)
      |     fprintf('%s -- Copyright %s Nexteer',NxtrConf,first)
      | else
      |     fprintf('%s -- %s%s- %s Nexteer',NxtrConf,char(169),first,last)
      | end
  Product2 : Product
  Bit1Sts : Outport
  wires:
  Constant1/1 -> Product2/1
  Constant2/1 -> Product2/2
  Product2/1 -> Bit1Sts/1

== system SF034A_AssiPahFwl/AssiPahFwl/AssiPahFwlPer1/Normal_Firewall_Operation/Set_Faults/Set AssiFwlFlt/If Action Subsystem3 ==
  Action Port : ActionPort  ActionType=else
  Constant1 : Constant  Value=0  OutDataTypeStr=uint8
      settings: AttributesFormatString=%<OutDataTypeStr>
  Constant2 : Constant  Value=BASASSIREACHED_CNT_U08
  CopyRight2 : Subsystem  Description=|  mask(Copyright Information){none=on}
      | Copyright info block.                                               
      |                                                                     
      | Place copyright information at the top of every subsystem in design.
      mask prompts: none "No parameters"
      mask help: Place copyright information at the top of every subsystem in design.
      mask Display:
      | NxtrConf = 'Nexteer Confidential';
      | 
      | sys = bdroot; %handle for the current model ("system")
      | first = get_param(sys,'Created');
      | first = first(end-3:end);  %year is last four digits
      | 
      | last = get_param(sys,'LastModifiedDate');
      | if isempty(last)
      |     last = datestr(now,'yyyy');
      | else
      |     last = last(end-3:end);
      | end
      | 
      | if strcmp(first,last)
      |     fprintf('%s -- Copyright %s Nexteer',NxtrConf,first)
      | else
      |     fprintf('%s -- %s%s- %s Nexteer',NxtrConf,char(169),first,last)
      | end
  Product2 : Product
  Bit1Sts : Outport
  wires:
  Product2/1 -> Bit1Sts/1
  Constant1/1 -> Product2/1
  Constant2/1 -> Product2/2

== system SF034A_AssiPahFwl/AssiPahFwl/AssiPahFwlPer1/Normal_Firewall_Operation/Debounce_BaseAssist_Overboundary/SetNtcSts/SetNtcSts/CopyRight2 ==

== system SF034A_AssiPahFwl/AssiPahFwl/AssiPahFwlPer1/Normal_Firewall_Operation/Debounce_BaseAssist_Overboundary/SetNtcSts1/SetNtcSts/CopyRight2 ==

== system SF034A_AssiPahFwl/AssiPahFwl/AssiPahFwlPer1/Normal_Firewall_Operation/Debounce_HiFreqAsst_Overboundary/SetNtcSts/SetNtcSts/CopyRight2 ==

== system SF034A_AssiPahFwl/AssiPahFwl/AssiPahFwlPer1/Normal_Firewall_Operation/Debounce_HiFreqAsst_Overboundary/SetNtcSts1/SetNtcSts/CopyRight2 ==
